simulink model "sim1"  (R2022a)
settings: Solver=VariableStepAuto  StartTime=0.0  StopTime=0.001  RelTol=1e-3
values from neighbouring files (symbols this model uses):
  v = 2.5    [test.m]    (also in test_Datacode.m = 5)
undefined symbols (not defined in the file or in its folder): fdesignblkfcn, gcbh
libraries: commchan3 x1, dsparch4 x1, simulink x1, dspfdesign x1, commrandsrc3 x1
settings Model: Creator=sky 2020  LastModifiedBy=sky 2020

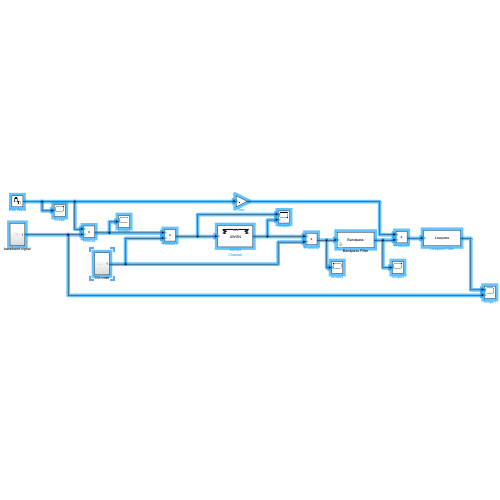
[thumbnail: Simulink's stored preview of the top-level diagram]
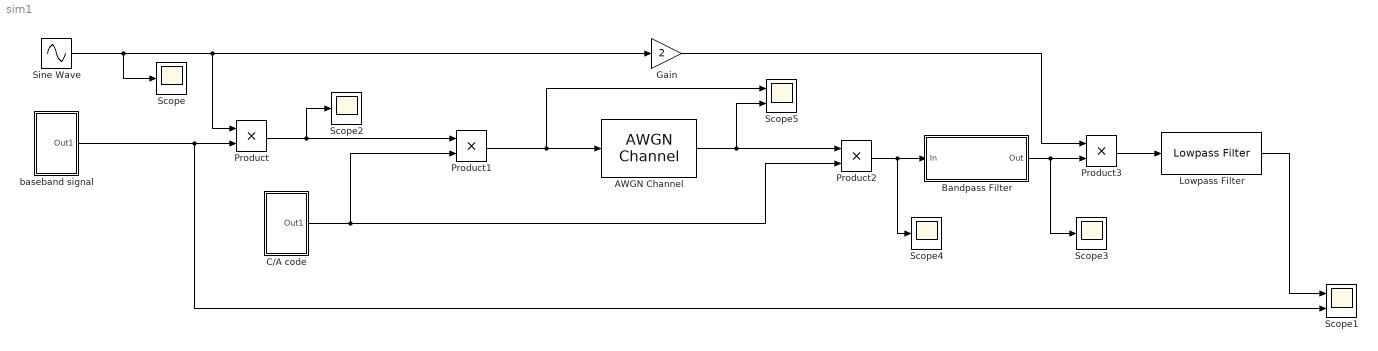
== system sim1 ==
  AWGN Channel : commchan3/AWGN Channel  InputProcessing=Columns as channels (frame based)  seed=67  noiseMode="Signal to noise ratio  (SNR)"  EbNodB=0  EsNodB=10  SNRdB=0  bitsPerSym=1  Ps=1  Tsym=1  variance=1
  Bandpass Filter : Subsystem  DialogController=fdesignblkfcn  InitFcn=fdesignblkfcn(gcbh, {'InitFcn'});  mask(Bandpass Filter){}
      mask help: Design a bandpass filter
      settings: CopyFcn=fdesignblkfcn(gcbh, {'CopyFcn'});
      mask Help: helpview(mapfilelocation('dsp'), 'dspbandpassfilter');
      mask Display: disp('Bandpass');
  C/A code : Subsystem
  Gain : Gain  Gain=2
  Lowpass Filter : dspfdesign/Lowpass Filter  FilterType=FIR  DesignForMinimumOrder=on  FilterOrder=50  PassbandFrequency=1.2e3  StopbandFrequency=2e3  PassbandRipple=0.1  StopbandAttenuation=60  InheritSampleRate=off  SampleRate=157.742e2  SimulateUsing=Interpreted execution  roundingMode=Floor  coeffsDataTypeStr=fixdt(1,16)
  Product{,1..3} (4 alike) : Product
  Scope{,2..4} (4 alike) : Scope
  Scope1 : Scope  NumInputPorts=2
  Scope5 : Scope  NumInputPorts=2
  Sine Wave : Sin  Frequency=2*pi*157.542e6  Phase=pi/2  SampleTime=1/(v*157.542e6)
  baseband signal : Subsystem
  wires:
  Gain/1 -> Product3/1
  Product3/1 -> Lowpass Filter/1
  Product/1 -> Scope2/1, Product1/1
  C/A code/1(Out1) -> Product2/2, Product1/2
  Product1/1 -> Scope5/1, AWGN Channel/1
  Sine Wave/1 -> Scope/1, Gain/1, Product/1
  baseband signal/1(Out1) -> Scope1/2, Product/2
  Lowpass Filter/1 -> Scope1/1
  Product2/1 -> Scope4/1, Bandpass Filter/1(In)
  AWGN Channel/1 -> Scope5/2, Product2/1
  Bandpass Filter/1(Out) -> Scope3/1, Product3/2

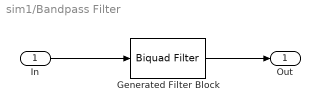
== system sim1/Bandpass Filter ==
  In : Inport
  Generated Filter Block : dsparch4/Biquad Filter  Tag=BlockMethodSubSystem  FilterSource=Dialog parameters  CoeffSource=Specify via dialog  FilterObject=BQF  IIRFiltStruct=Direct form II  BiQuadCoeffs=[0.00380302990539071279 0 -0.00380302990539071279 1 1.61904346999335025 0.998458791755205466;0.00222628283797649028 0 -0.00222628283797649028 1 1.61451631506587345 0.998450612907040735;0.851459124863951367 0 -0.851459124863951367 1 1.61553762151329305 0.996911779330365899]  ScaleValues=[0.000919689030413472098;1;1;1]  IC=0  ICnum=0  ICden=0  a0Flag=Warning  optimizeScaleValues=off  ScaleValueMode=Specify via input port (g)  InputProcessing=Columns as channels (frame based)  roundingMode=Floor  overflowMode=off  scaleValueFracLength=14  denProdOutputFracLength=30  denAccumFracLength=30  secondMemoryFracLength=15
  Out : Outport  VectorParamsAs1DForOutWhenUnconnected=off
  wires:
  In/1 -> Generated Filter Block/1
  Generated Filter Block/1 -> Out/1

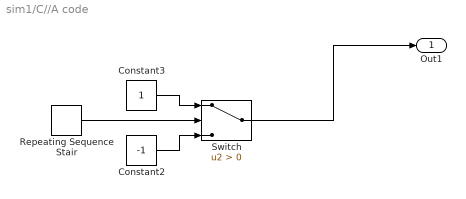
== system sim1/C//A code ==
  Constant2 : Constant  Value=-1
  Constant3 : Constant
  Repeating Sequence Stair : simulink/Sources/Repeating Sequence Stair  OutValues=ca1  tsamp=1e-3/1023  OutMin=[]  OutMax=[]  OutDataTypeStr=double  OutputDataTypeScalingMode=double  OutDataType=fixdt(0,8)  ConRadixGroup=Best Precision: Vector-wise  OutScaling=2^-12
  Switch : Switch  Criteria=u2 > Threshold  SaturateOnIntegerOverflow=off  InputSameDT=off
  Out1 : Outport
  wires:
  Repeating Sequence Stair/1 -> Switch/2
  Constant2/1 -> Switch/3
  Constant3/1 -> Switch/1
  Switch/1 -> Out1/1

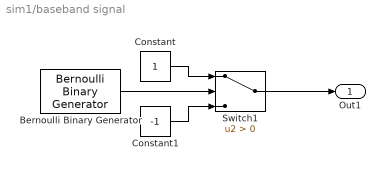
== system sim1/baseband signal ==
  Bernoulli Binary Generator : commrandsrc3/Bernoulli Binary Generator  ProbabilityOfZero=0.5  SeedSource=Auto  Seed=0  SampleTime=1/1e3  SamplesPerFrame=1  OutputDataType=double  SimulateUsing=Interpreted execution
  Constant : Constant
  Constant1 : Constant  Value=-1
  Switch1 : Switch  Criteria=u2 > Threshold  SaturateOnIntegerOverflow=off  InputSameDT=off
  Out1 : Outport
  wires:
  Constant1/1 -> Switch1/3
  Constant/1 -> Switch1/1
  Bernoulli Binary Generator/1 -> Switch1/2
  Switch1/1 -> Out1/1
